simulink model "inverse_dynamic_with_pid"  (R2018a)
settings: Solver=ode45  StartTime=0.0  StopTime=3  RelTol=1e-3
libraries: simulink x6
settings Model: Creator=JORDAN  LastModifiedBy=JORDAN
settings DebuggingCC: LibraryContextMissingDiagnostic=warning
settings SFSimCC: SimUseLocalCustomCode=on
settings RTWCC: RTWUseLocalCustomCode=on

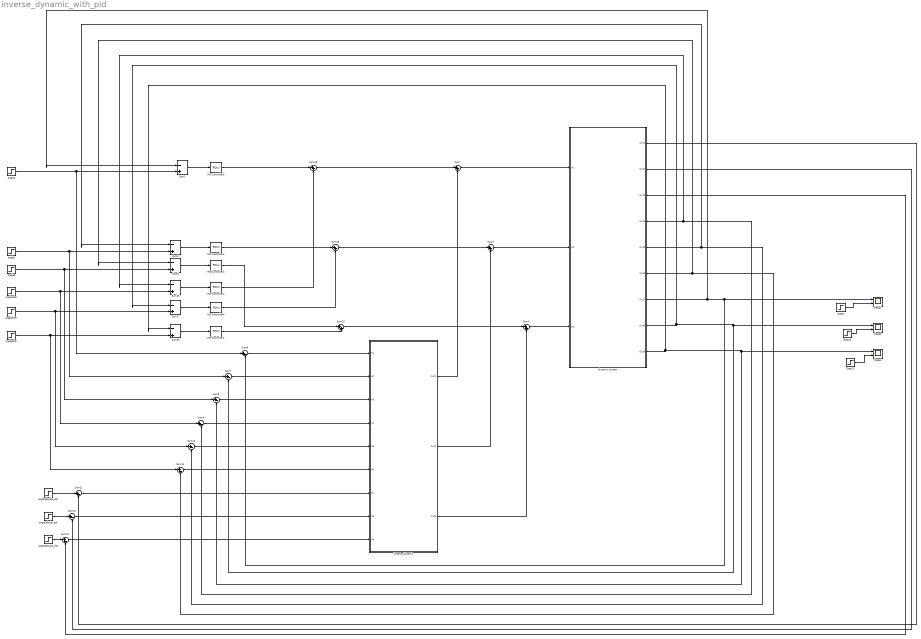
== system inverse_dynamic_with_pid ==
  PID Controller1 : simulink/Continuous/PID Controller  Controller=PD  Form=Parallel  TimeDomain=Continuous-time  SampleTime=-1  IntegratorMethod=Forward Euler  FilterMethod=Forward Euler  ControllerParametersSource=internal  P=75000  I=1  D=6000  UseFilter=on  N=7500  TunerSelectOption=Transfer Function Based (PID Tuner App)  InitialConditionSource=internal  InitialConditionForIntegrator=0  InitialConditionForFilter=0  DifferentiatorICPrevScaledInput=0  ExternalReset=none  TrackingMode=off  Kt=1  LimitOutput=off  UpperSaturationLimit=inf  LowerSaturationLimit=-inf  LinearizeAsGain=on  AntiWindupMode=none  Kb=1  POutMin=[]  POutMax=[]  IOutMin=[]  IOutMax=[]  DOutMin=[]  DOutMax=[]  NOutMin=[]  NOutMax=[]  SumOutMin=[]  SumOutMax=[]  SaturationOutMin=[]  SaturationOutMax=[]  PParamMin=[]  PParamMax=[]  IParamMin=[]  IParamMax=[]  DParamMin=[]  DParamMax=[]  NParamMin=[]  NParamMax=[]  KbParamMin=[]  KbParamMax=[]  KtParamMin=[]  KtParamMax=[]  KbOutMin=[]  KbOutMax=[]  KtOutMin=[]  KtOutMax=[]  IntegratorOutMin=[]  IntegratorOutMax=[]  FilterOutMin=[]  FilterOutMax=[]  SumI1OutMin=[]  SumI1OutMax=[]  SumI2OutMin=[]  SumI2OutMax=[]  SumI3OutMin=[]  SumI3OutMax=[]  SumDOutMin=[]  SumDOutMax=[]  DifferentiatorOutMin=[]  DifferentiatorOutMax=[]  FilterDiffOutCoefMin=[]  FilterDiffOutCoefMax=[]  ReciprocalOutMin=[]  ReciprocalOutMax=[]  SumDenOutMin=[]  SumDenOutMax=[]  SumNumOutMin=[]  SumNumOutMax=[]  DivideOutMin=[]  DivideOutMax=[]  IntegratorContinuousStateAttributes=''  IntegratorStateMustResolveToSignalObject=off  IntegratorRTWStateStorageClass=Auto  FilterContinuousStateAttributes=''  FilterStateMustResolveToSignalObject=off  FilterRTWStateStorageClass=Auto
  PID Controller2 : simulink/Continuous/PID Controller  Controller=PD  Form=Parallel  TimeDomain=Continuous-time  SampleTime=-1  IntegratorMethod=Forward Euler  FilterMethod=Forward Euler  ControllerParametersSource=internal  P=6000  I=1  D=0  UseFilter=on  N=100  TunerSelectOption=Transfer Function Based (PID Tuner App)  InitialConditionSource=internal  InitialConditionForIntegrator=0  InitialConditionForFilter=0  DifferentiatorICPrevScaledInput=0  ExternalReset=none  TrackingMode=off  Kt=1  LimitOutput=off  UpperSaturationLimit=inf  LowerSaturationLimit=-inf  LinearizeAsGain=on  AntiWindupMode=none  Kb=1  POutMin=[]  POutMax=[]  IOutMin=[]  IOutMax=[]  DOutMin=[]  DOutMax=[]  NOutMin=[]  NOutMax=[]  SumOutMin=[]  SumOutMax=[]  SaturationOutMin=[]  SaturationOutMax=[]  PParamMin=[]  PParamMax=[]  IParamMin=[]  IParamMax=[]  DParamMin=[]  DParamMax=[]  NParamMin=[]  NParamMax=[]  KbParamMin=[]  KbParamMax=[]  KtParamMin=[]  KtParamMax=[]  KbOutMin=[]  KbOutMax=[]  KtOutMin=[]  KtOutMax=[]  IntegratorOutMin=[]  IntegratorOutMax=[]  FilterOutMin=[]  FilterOutMax=[]  SumI1OutMin=[]  SumI1OutMax=[]  SumI2OutMin=[]  SumI2OutMax=[]  SumI3OutMin=[]  SumI3OutMax=[]  SumDOutMin=[]  SumDOutMax=[]  DifferentiatorOutMin=[]  DifferentiatorOutMax=[]  FilterDiffOutCoefMin=[]  FilterDiffOutCoefMax=[]  ReciprocalOutMin=[]  ReciprocalOutMax=[]  SumDenOutMin=[]  SumDenOutMax=[]  SumNumOutMin=[]  SumNumOutMax=[]  DivideOutMin=[]  DivideOutMax=[]  IntegratorContinuousStateAttributes=''  IntegratorStateMustResolveToSignalObject=off  IntegratorRTWStateStorageClass=Auto  FilterContinuousStateAttributes=''  FilterStateMustResolveToSignalObject=off  FilterRTWStateStorageClass=Auto
  PID Controller3 : simulink/Continuous/PID Controller  Controller=PD  Form=Parallel  TimeDomain=Continuous-time  SampleTime=-1  IntegratorMethod=Forward Euler  FilterMethod=Forward Euler  ControllerParametersSource=internal  P=150  I=1  D=0  UseFilter=on  N=100  TunerSelectOption=Transfer Function Based (PID Tuner App)  InitialConditionSource=internal  InitialConditionForIntegrator=0  InitialConditionForFilter=0  DifferentiatorICPrevScaledInput=0  ExternalReset=none  TrackingMode=off  Kt=1  LimitOutput=off  UpperSaturationLimit=inf  LowerSaturationLimit=-inf  LinearizeAsGain=on  AntiWindupMode=none  Kb=1  POutMin=[]  POutMax=[]  IOutMin=[]  IOutMax=[]  DOutMin=[]  DOutMax=[]  NOutMin=[]  NOutMax=[]  SumOutMin=[]  SumOutMax=[]  SaturationOutMin=[]  SaturationOutMax=[]  PParamMin=[]  PParamMax=[]  IParamMin=[]  IParamMax=[]  DParamMin=[]  DParamMax=[]  NParamMin=[]  NParamMax=[]  KbParamMin=[]  KbParamMax=[]  KtParamMin=[]  KtParamMax=[]  KbOutMin=[]  KbOutMax=[]  KtOutMin=[]  KtOutMax=[]  IntegratorOutMin=[]  IntegratorOutMax=[]  FilterOutMin=[]  FilterOutMax=[]  SumI1OutMin=[]  SumI1OutMax=[]  SumI2OutMin=[]  SumI2OutMax=[]  SumI3OutMin=[]  SumI3OutMax=[]  SumDOutMin=[]  SumDOutMax=[]  DifferentiatorOutMin=[]  DifferentiatorOutMax=[]  FilterDiffOutCoefMin=[]  FilterDiffOutCoefMax=[]  ReciprocalOutMin=[]  ReciprocalOutMax=[]  SumDenOutMin=[]  SumDenOutMax=[]  SumNumOutMin=[]  SumNumOutMax=[]  DivideOutMin=[]  DivideOutMax=[]  IntegratorContinuousStateAttributes=''  IntegratorStateMustResolveToSignalObject=off  IntegratorRTWStateStorageClass=Auto  FilterContinuousStateAttributes=''  FilterStateMustResolveToSignalObject=off  FilterRTWStateStorageClass=Auto
  PID Controller4 : simulink/Continuous/PID Controller  Controller=PD  Form=Parallel  TimeDomain=Continuous-time  SampleTime=-1  IntegratorMethod=Forward Euler  FilterMethod=Forward Euler  ControllerParametersSource=internal  P=1  I=1  D=0  UseFilter=on  N=100  TunerSelectOption=Transfer Function Based (PID Tuner App)  InitialConditionSource=internal  InitialConditionForIntegrator=0  InitialConditionForFilter=0  DifferentiatorICPrevScaledInput=0  ExternalReset=none  TrackingMode=off  Kt=1  LimitOutput=off  UpperSaturationLimit=inf  LowerSaturationLimit=-inf  LinearizeAsGain=on  AntiWindupMode=none  Kb=1  POutMin=[]  POutMax=[]  IOutMin=[]  IOutMax=[]  DOutMin=[]  DOutMax=[]  NOutMin=[]  NOutMax=[]  SumOutMin=[]  SumOutMax=[]  SaturationOutMin=[]  SaturationOutMax=[]  PParamMin=[]  PParamMax=[]  IParamMin=[]  IParamMax=[]  DParamMin=[]  DParamMax=[]  NParamMin=[]  NParamMax=[]  KbParamMin=[]  KbParamMax=[]  KtParamMin=[]  KtParamMax=[]  KbOutMin=[]  KbOutMax=[]  KtOutMin=[]  KtOutMax=[]  IntegratorOutMin=[]  IntegratorOutMax=[]  FilterOutMin=[]  FilterOutMax=[]  SumI1OutMin=[]  SumI1OutMax=[]  SumI2OutMin=[]  SumI2OutMax=[]  SumI3OutMin=[]  SumI3OutMax=[]  SumDOutMin=[]  SumDOutMax=[]  DifferentiatorOutMin=[]  DifferentiatorOutMax=[]  FilterDiffOutCoefMin=[]  FilterDiffOutCoefMax=[]  ReciprocalOutMin=[]  ReciprocalOutMax=[]  SumDenOutMin=[]  SumDenOutMax=[]  SumNumOutMin=[]  SumNumOutMax=[]  DivideOutMin=[]  DivideOutMax=[]  IntegratorContinuousStateAttributes=''  IntegratorStateMustResolveToSignalObject=off  IntegratorRTWStateStorageClass=Auto  FilterContinuousStateAttributes=''  FilterStateMustResolveToSignalObject=off  FilterRTWStateStorageClass=Auto
  PID Controller5 : simulink/Continuous/PID Controller  Controller=PD  Form=Parallel  TimeDomain=Continuous-time  SampleTime=-1  IntegratorMethod=Forward Euler  FilterMethod=Forward Euler  ControllerParametersSource=internal  P=1  I=1  D=0  UseFilter=on  N=100  TunerSelectOption=Transfer Function Based (PID Tuner App)  InitialConditionSource=internal  InitialConditionForIntegrator=0  InitialConditionForFilter=0  DifferentiatorICPrevScaledInput=0  ExternalReset=none  TrackingMode=off  Kt=1  LimitOutput=off  UpperSaturationLimit=inf  LowerSaturationLimit=-inf  LinearizeAsGain=on  AntiWindupMode=none  Kb=1  POutMin=[]  POutMax=[]  IOutMin=[]  IOutMax=[]  DOutMin=[]  DOutMax=[]  NOutMin=[]  NOutMax=[]  SumOutMin=[]  SumOutMax=[]  SaturationOutMin=[]  SaturationOutMax=[]  PParamMin=[]  PParamMax=[]  IParamMin=[]  IParamMax=[]  DParamMin=[]  DParamMax=[]  NParamMin=[]  NParamMax=[]  KbParamMin=[]  KbParamMax=[]  KtParamMin=[]  KtParamMax=[]  KbOutMin=[]  KbOutMax=[]  KtOutMin=[]  KtOutMax=[]  IntegratorOutMin=[]  IntegratorOutMax=[]  FilterOutMin=[]  FilterOutMax=[]  SumI1OutMin=[]  SumI1OutMax=[]  SumI2OutMin=[]  SumI2OutMax=[]  SumI3OutMin=[]  SumI3OutMax=[]  SumDOutMin=[]  SumDOutMax=[]  DifferentiatorOutMin=[]  DifferentiatorOutMax=[]  FilterDiffOutCoefMin=[]  FilterDiffOutCoefMax=[]  ReciprocalOutMin=[]  ReciprocalOutMax=[]  SumDenOutMin=[]  SumDenOutMax=[]  SumNumOutMin=[]  SumNumOutMax=[]  DivideOutMin=[]  DivideOutMax=[]  IntegratorContinuousStateAttributes=''  IntegratorStateMustResolveToSignalObject=off  IntegratorRTWStateStorageClass=Auto  FilterContinuousStateAttributes=''  FilterStateMustResolveToSignalObject=off  FilterRTWStateStorageClass=Auto
  PID Controller6 : simulink/Continuous/PID Controller  Controller=PD  Form=Parallel  TimeDomain=Continuous-time  SampleTime=-1  IntegratorMethod=Forward Euler  FilterMethod=Forward Euler  ControllerParametersSource=internal  P=337900  I=1  D=19000  UseFilter=on  N=6170  TunerSelectOption=Transfer Function Based (PID Tuner App)  InitialConditionSource=internal  InitialConditionForIntegrator=0  InitialConditionForFilter=0  DifferentiatorICPrevScaledInput=0  ExternalReset=none  TrackingMode=off  Kt=1  LimitOutput=off  UpperSaturationLimit=inf  LowerSaturationLimit=-inf  LinearizeAsGain=on  AntiWindupMode=none  Kb=1  POutMin=[]  POutMax=[]  IOutMin=[]  IOutMax=[]  DOutMin=[]  DOutMax=[]  NOutMin=[]  NOutMax=[]  SumOutMin=[]  SumOutMax=[]  SaturationOutMin=[]  SaturationOutMax=[]  PParamMin=[]  PParamMax=[]  IParamMin=[]  IParamMax=[]  DParamMin=[]  DParamMax=[]  NParamMin=[]  NParamMax=[]  KbParamMin=[]  KbParamMax=[]  KtParamMin=[]  KtParamMax=[]  KbOutMin=[]  KbOutMax=[]  KtOutMin=[]  KtOutMax=[]  IntegratorOutMin=[]  IntegratorOutMax=[]  FilterOutMin=[]  FilterOutMax=[]  SumI1OutMin=[]  SumI1OutMax=[]  SumI2OutMin=[]  SumI2OutMax=[]  SumI3OutMin=[]  SumI3OutMax=[]  SumDOutMin=[]  SumDOutMax=[]  DifferentiatorOutMin=[]  DifferentiatorOutMax=[]  FilterDiffOutCoefMin=[]  FilterDiffOutCoefMax=[]  ReciprocalOutMin=[]  ReciprocalOutMax=[]  SumDenOutMin=[]  SumDenOutMax=[]  SumNumOutMin=[]  SumNumOutMax=[]  DivideOutMin=[]  DivideOutMax=[]  IntegratorContinuousStateAttributes=''  IntegratorStateMustResolveToSignalObject=off  IntegratorRTWStateStorageClass=Auto  FilterContinuousStateAttributes=''  FilterStateMustResolveToSignalObject=off  FilterRTWStateStorageClass=Auto
  Step10 : Step  Time=0  SampleTime=0
  Step11 : Step  Time=0  SampleTime=0
  Step9 : Step  Time=0  SampleTime=0
  Sum{,3..4,18..20} (6 alike) : Sum  Inputs=|++
  Sum{1..2,5,15..17} (6 alike) : Sum  Inputs=|-+
  Sum{6..14} (9 alike) : Sum  Inputs=|+-
  angle1 : Step  SampleTime=0
  angle1dot : Step  Time=0  SampleTime=0
  angle1double_dot : Step  Time=0  SampleTime=0
  angle2 : Step  SampleTime=0
  angle2dot : Step  Time=0  SampleTime=0
  angle2doule_dot : Step  Time=0  SampleTime=0
  angle3 : Step  SampleTime=0
  angle3dot : Step  Time=0  SampleTime=0
  angle3double_dot : Step  Time=0  SampleTime=0
  dynamic system : Subsystem
  inverse_dynamic : Subsystem
  theta1 : Scope  NumInputPorts=2
  theta2 : Scope  NumInputPorts=2
  theta3 : Scope  NumInputPorts=2
  wires:
  inverse_dynamic/1(Out1) -> Sum/2
  inverse_dynamic/2(Out2) -> Sum3/2
  inverse_dynamic/3(Out3) -> Sum4/2
  angle1/1 -> Sum6/1, Sum1/2
  angle3/1 -> Sum5/2, Sum8/1
  angle2dot/1 -> Sum17/2, Sum14/1
  angle3dot/1 -> Sum12/1, Sum15/2
  angle1dot/1 -> Sum16/2, Sum9/1
  angle2/1 -> Sum2/2, Sum7/1
  angle1double_dot/1 -> Sum11/1
  angle2doule_dot/1 -> Sum10/1
  angle3double_dot/1 -> Sum13/1
  Sum6/1 -> inverse_dynamic/1(In1)
  Sum7/1 -> inverse_dynamic/2(In2)
  Sum8/1 -> inverse_dynamic/3(In3)
  Sum9/1 -> inverse_dynamic/4(In4)
  Sum14/1 -> inverse_dynamic/5(In5)
  Sum12/1 -> inverse_dynamic/6(In6)
  Sum11/1 -> inverse_dynamic/7(In7)
  Sum10/1 -> inverse_dynamic/8(In8)
  Sum13/1 -> inverse_dynamic/9(In9)
  Sum1/1 -> PID Controller5/1
  Sum2/1 -> PID Controller2/1
  Sum5/1 -> PID Controller3/1
  dynamic system/8(Out8) -> Sum17/1, theta2/1, Sum7/2
  dynamic system/9(Out9) -> theta3/1, Sum8/2, Sum15/1
  dynamic system/7(Out7) -> Sum1/1, theta1/1, Sum6/2
  dynamic system/5(Out5) -> Sum2/1, Sum14/2
  dynamic system/2(Out2) -> Sum10/2
  dynamic system/4(Out4) -> Sum16/1, Sum9/2
  Sum4/1 -> dynamic system/3(In3)
  dynamic system/3(Out3) -> Sum13/2
  dynamic system/6(Out6) -> Sum5/1, Sum12/2
  dynamic system/1(Out1) -> Sum11/2
  Sum3/1 -> dynamic system/2(In2)
  Sum/1 -> dynamic system/1(In1)
  Sum15/1 -> PID Controller1/1
  Sum17/1 -> PID Controller6/1
  Sum16/1 -> PID Controller4/1
  PID Controller5/1 -> Sum19/1
  PID Controller4/1 -> Sum19/2
  PID Controller2/1 -> Sum18/1
  PID Controller6/1 -> Sum18/2
  PID Controller3/1 -> Sum20/1
  PID Controller1/1 -> Sum20/2
  Sum19/1 -> Sum/1
  Sum18/1 -> Sum3/1
  Sum20/1 -> Sum4/1
  Step9/1 -> theta1/2
  Step10/1 -> theta2/2
  Step11/1 -> theta3/2

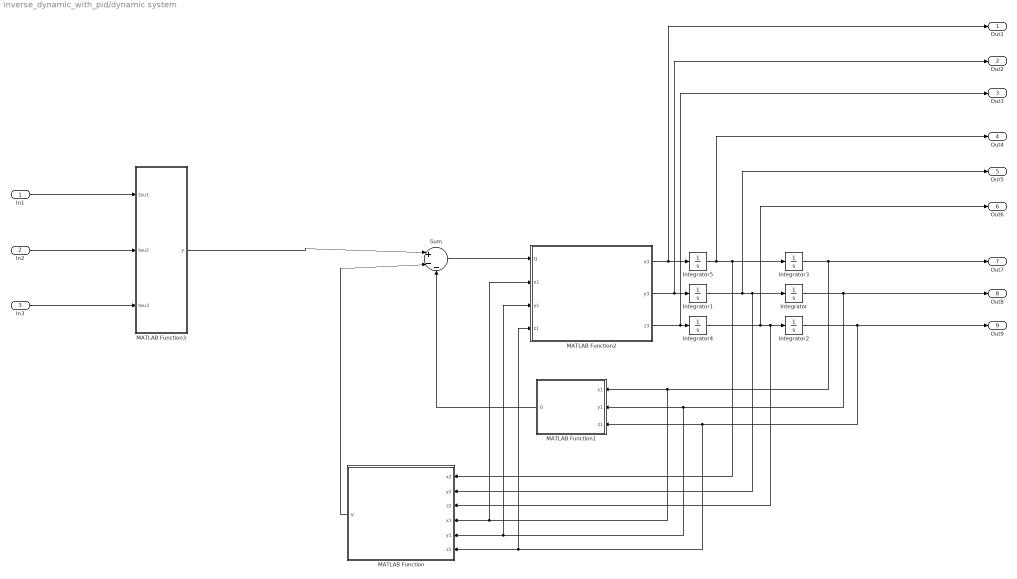
== system inverse_dynamic_with_pid/dynamic system ==
  In1 : Inport
  In2 : Inport  Port=2
  In3 : Inport  Port=3
  Integrator{,2..5} (5 alike) : Integrator
  Integrator1 : Integrator  InitialCondition=0.0000001
  MATLAB Function : MATLAB Function  TreatAsAtomicUnit=on
  MATLAB Function1 : MATLAB Function  TreatAsAtomicUnit=on
  MATLAB Function2 : MATLAB Function  TreatAsAtomicUnit=on
  MATLAB Function3 : MATLAB Function  TreatAsAtomicUnit=on
  Sum : Sum  Inputs=|+--
  Out1 : Outport
  Out2 : Outport  Port=2
  Out3 : Outport  Port=3
  Out4 : Outport  Port=4
  Out5 : Outport  Port=5
  Out6 : Outport  Port=6
  Out7 : Outport  Port=7
  Out8 : Outport  Port=8
  Out9 : Outport  Port=9
  wires:
  Integrator5/1 -> Out4/1, MATLAB Function/1(x2), Integrator3/1
  Integrator1/1 -> Out5/1, Integrator/1, MATLAB Function/2(y2)
  Integrator3/1 -> Out7/1, MATLAB Function2/2(x1), MATLAB Function/4(x1), MATLAB Function1/1(x1)
  MATLAB Function2/3(z3) -> Out3/1, Integrator4/1
  Integrator4/1 -> Out6/1, MATLAB Function/3(z2), Integrator2/1
  MATLAB Function2/2(y3) -> Out2/1, Integrator1/1
  Integrator/1 -> Out8/1, MATLAB Function2/3(y1), MATLAB Function/5(y1), MATLAB Function1/2(y1)
  MATLAB Function/1(V) -> Sum/2
  MATLAB Function2/1(x3) -> Out1/1, Integrator5/1
  MATLAB Function1/1(G) -> Sum/3
  In2/1 -> MATLAB Function3/2(tau2)
  In1/1 -> MATLAB Function3/1(tau1)
  Sum/1 -> MATLAB Function2/1(Q)
  Integrator2/1 -> Out9/1, MATLAB Function2/4(z1), MATLAB Function/6(z1), MATLAB Function1/3(z1)
  MATLAB Function3/1(y) -> Sum/1
  In3/1 -> MATLAB Function3/3(tau3)

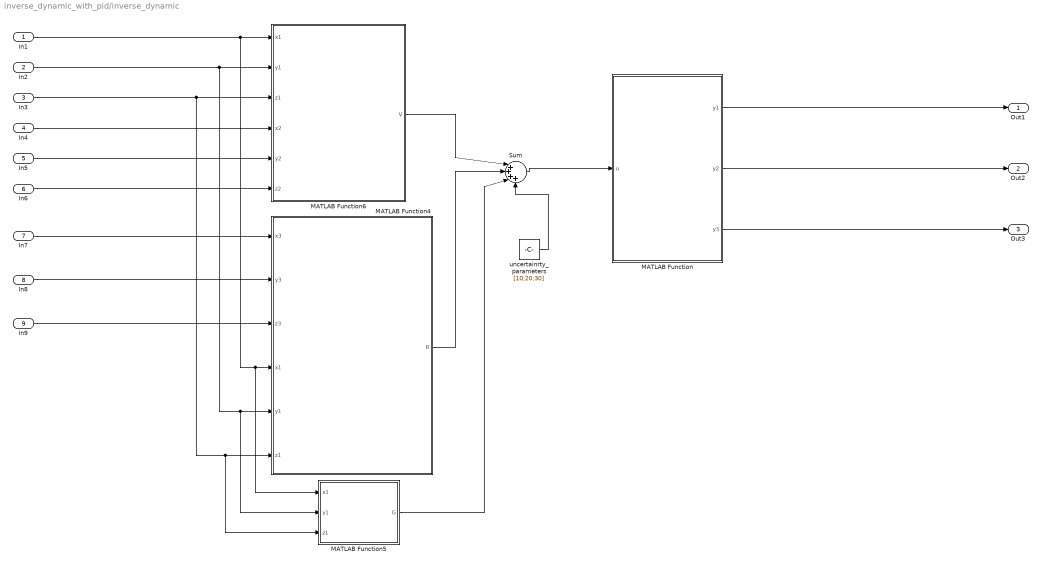
== system inverse_dynamic_with_pid/inverse_dynamic ==
  In1 : Inport
  In2 : Inport  Port=2
  In3 : Inport  Port=3
  In4 : Inport  Port=4
  In5 : Inport  Port=5
  In6 : Inport  Port=6
  In7 : Inport  Port=7
  In8 : Inport  Port=8
  In9 : Inport  Port=9
  MATLAB Function : MATLAB Function  TreatAsAtomicUnit=on
  MATLAB Function4 : MATLAB Function  TreatAsAtomicUnit=on
  MATLAB Function5 : MATLAB Function  TreatAsAtomicUnit=on
  MATLAB Function6 : MATLAB Function  TreatAsAtomicUnit=on
  Sum : Sum  Inputs=|++++
  uncertainrty_parameters : Constant  Value=[10;20;30]
  Out1 : Outport
  Out2 : Outport  Port=2
  Out3 : Outport  Port=3
  wires:
  MATLAB Function/1(y1) -> Out1/1
  MATLAB Function/2(y2) -> Out2/1
  In1/1 -> MATLAB Function5/1(x1), MATLAB Function4/4(x1), MATLAB Function6/1(x1)
  In2/1 -> MATLAB Function5/2(y1), MATLAB Function4/5(y1), MATLAB Function6/2(y1)
  In3/1 -> MATLAB Function5/3(z1), MATLAB Function4/6(z1), MATLAB Function6/3(z1)
  MATLAB Function4/1(R) -> Sum/2
  MATLAB Function6/1(V) -> Sum/1
  MATLAB Function5/1(G) -> Sum/3
  Sum/1 -> MATLAB Function/1(u)
  In5/1 -> MATLAB Function6/5(y2)
  In6/1 -> MATLAB Function6/6(z2)
  MATLAB Function/3(y3) -> Out3/1
  In4/1 -> MATLAB Function6/4(x2)
  In7/1 -> MATLAB Function4/1(x3)
  In9/1 -> MATLAB Function4/3(z3)
  In8/1 -> MATLAB Function4/2(y3)
  uncertainrty_parameters/1 -> Sum/4

== matlab function inverse_dynamic_with_pid/dynamic system/MATLAB Function ==
  data: x2 input; V output size=3*1; y2 input; z2 input; x1 input; y1 input; z1 input
function V = vmatrix(x2,y2,z2,x1,y1,z1)
m2=3; 
m3=2;
l2=5; 
l3=3;
r=10;
V=[(-0.25*m3*(r^2)*sin(y1)*cos(y1)*x2*z2)-((1/6)*m2*l2^2*cos(y1)*sin(y1)*x2*y2)+((2/3)*m3*l3^2*cos(y1)*cos(z1)*sin(z1-y1)*x2*y2)+(0.5*m3*(r^2)*sin(y1-z1)*cos(y1-z1)*x2*y2)+((3/4)*m2*(r^2)*sin(y1)*cos(y1)*x2*y2)+((1/6)*m3*l3^2*sin(y1)*sin(z1-x1)*x2*y2)+(0.5*m3*l3^2*sin(y1)*sin(z1)*sin(z1-y1)*x2*y2)+(0.5*m3*l2*l3*cos(y1)*cos(y1-z1)*x2)+(m3*l2*l3*sin(y1)*sin(y1)*sin(z1)*x2*y2)-(0.25*m2*(r^2)*cos(y1)*sin(y1)*x2*y2)-(m3*l2*l3*cos(y1)*sin(y1)*cos(z1)*x2*y2)-(0.5*m2*l2^2*cos(y1)*sin(y1)*x2*y2)+(m3*l2*l3*cos(y1)*sin(z1-y1)*x2*y2)+(m3*l2^2*cos(y1)*cos(y1)*x2)+(2*m3*l2^2*cos(y1)*sin(y1)*x2*y2) ; 
    (-0.25*m2*(r^2)*cos(y1)*sin(y1)*(x2^2))+((1/12)*m2*l2^2*sin(y1)*cos(y1)*(x2^2))+(0.25*m3*(r^2)*cos(y1-z1)*sin(z1-y1)*(x2^2))-((1/3)*m3*l3^2*cos(y1-z1)*sin(z1-y1)*(x2^2))-(0.25*m3*l3^2*z2)+(0.5*m3*l3*l2*cos(y1)*cos(z1-y1)*(x2^2))-(0.5*m3*l3*l2*sin(z1)*(y2^2))+(0.25*m2*l2^2*sin(y1)*cos(y1)*(x2^2))+(0.5*m3*l3*l2*sin(z1)*cos(y1-z1)*(x2^2))+(0.5*m3*l3*l2*sin(z1)*(z2^2))+(0.5*m3*l3*l2*sin(z1)*(y2^2))-(m3*l3*l2*sin(z1)*y2*z2)+(m3*l2^2*cos(y1)*sin(y1)*cos(z1-y1)*(x2^2))-(0.5*m3*l3*l2*cos(z1)*cos(y1-z1)*sin(z1-y1)*(x2^2))+(m3*l2^2*cos(y1)*cos(z1)*cos(z1-y1)*(x2^2)) ; 
    (-0.25*m3*(r^2)*cos(y1-z1)*sin(z1-y1)*(x2^2))+((1/3)*m3*l3^2*cos(y1-z1)*sin(z1-y1)*(x2^2))+(0.25*m3*l3^2*z2)-(0.5*m3*l3*l2*cos(y1)*cos(z1-y1)*(x2^2))+(0.5*m3*l3*l2*sin(z1)*(y2^2))];

== matlab function inverse_dynamic_with_pid/inverse_dynamic/MATLAB Function ==
  data: u input; y1 output; y2 output; y3 output
function [y1,y2,y3] = tau_matrix(u)

y1=u(1,1);
y2=u(2,1);
y3=u(3,1);

== matlab function inverse_dynamic_with_pid/dynamic system/MATLAB Function1 ==
  data: x1 input; G output; y1 input; z1 input
function G = gravity(x1,y1,z1)
g=10;
m2=3;
m3=2;
l2=5;
l3=3;
r=10;
G=[0 ; (-0.5*m3*l2*cos(y1-z1)*g)-(0.5*m2*l2*cos(y1)*g)+(m3*l2*sin(z1)*sin(y1-z1)*g) ; (0.5*m3*l3*cos(y1-z1)*g)]

== matlab function inverse_dynamic_with_pid/dynamic system/MATLAB Function2 ==
  data: Q input; x3 output; y3 output; z3 output; x1 input; y1 input; z1 input
function  [x3,y3,z3]= mass_matrix(Q,x1,y1,z1)
m1=5;
m2=3;
m3=2;
l2=5;
l3=3;
r=10;
p=[(0.25*m2*(r^2)*((2*sin(y1)*sin(y1))+(cos(y1)*cos(y1))))+(0.25*m3*(r^2)*((2*sin(z1-y1)*sin(z1-y1))+(cos(z1-y1)*cos(z1-y1))))+((1/12)*m3*sin(y1)*sin(z1)*cos(y1-z1)*(l2^2+3*l3^2))+((1/6)*m3*l3*cos(y1)*cos(y1-z1)*(2*l3*cos(z1)+3*l2))+(0.5*m1*r)+((1/3)*m2*l2^2*cos(y1)*cos(y1)) 0 0 ; 
0 ((1/12)*m2*((3*r^2)+l2^2))+(0.25*m3*(r^2+l3^2))+(m3*l3*l2*cos(z1)+(l2^2*(0.25*m2+m3))) (-(1/12)*m3*((3*r^2)+4*l3^2))-(0.5*m3*l3*l2*cos(z1)) ; 
0 (-(1/12)*m3*(3*r^2+4*l3^2))-(0.5*m3*l3*l2*cos(z1)) ((1/12)*m3*(3*r^2+l3^2))]
R=inv(p)*Q
x3=R(1,1);
y3=R(2,1);
z3=R(3,1);

== matlab function inverse_dynamic_with_pid/inverse_dynamic/MATLAB Function4 ==
  data: x3 input; y3 input; z3 input; R output; x1 input; y1 input; z1 input
function R = mass_matrix(x3,y3,z3,x1,y1,z1)
m1=5;
m2=3;
m3=2;
l2=5;
l3=3;
r=10;
p=[(0.25*m2*(r^2)*((2*sin(y1)*sin(y1))+(cos(y1)*cos(y1))))+(0.25*m3*(r^2)*((2*sin(z1-y1)*sin(z1-y1))+(cos(z1-y1)*cos(z1-y1))))+((1/12)*m3*sin(y1)*sin(z1)*cos(y1-z1)*(l2^2+3*l3^2))+((1/6)*m3*l3*cos(y1)*cos(y1-z1)*(2*l3*cos(z1)+3*l2))+(0.5*m1*r)+((1/3)*m2*l2^2*cos(y1)*cos(y1)) 0 0 ; 
0 ((1/12)*m2*((3*r^2)+l2^2))+(0.25*m3*(r^2+l3^2))+(m3*l3*l2*cos(z1)+(l2^2*(0.25*m2+m3))) (-(1/12)*m3*((3*r^2)+4*l3^2))-(0.5*m3*l3*l2*cos(z1)) ; 
0 (-(1/12)*m3*(3*r^2+4*l3^2))-(0.5*m3*l3*l2*cos(z1)) ((1/12)*m3*(3*r^2+l3^2))]
n=[x3;y3;z3];
R=p*n

== matlab function inverse_dynamic_with_pid/inverse_dynamic/MATLAB Function5 ==
  data: x1 input; G output; y1 input; z1 input
function G = gravity(x1,y1,z1)
g=10;
m2=3;
m3=2;
l2=5;
l3=3;
r=10;
G=[0 ; (-0.5*m3*l2*cos(y1-z1)*g)-(0.5*m2*l2*cos(y1)*g)+(m3*l2*sin(z1)*sin(y1-z1)*g) ; (0.5*m3*l3*cos(y1-z1)*g)]

== matlab function inverse_dynamic_with_pid/dynamic system/MATLAB Function3 ==
  data: tau1 input; y output; tau2 input; tau3 input
function y = tau_matix(tau1,tau2,tau3)
y=[tau1;tau2;tau3];

== matlab function inverse_dynamic_with_pid/inverse_dynamic/MATLAB Function6 ==
  data: x1 input; y1 input; z1 input; x2 input; V output size=3*1; y2 input; z2 input
function V = vmatrix(x1,y1,z1,x2,y2,z2)
m2=3; 
m3=2;
l2=5; 
l3=3;
r=10;
V=[(-0.25*m3*(r^2)*sin(y1)*cos(y1)*x2*z2)-((1/6)*m2*l2^2*cos(y1)*sin(y1)*x2*y2)+((2/3)*m3*l3^2*cos(y1)*cos(z1)*sin(z1-y1)*x2*y2)+(0.5*m3*(r^2)*sin(y1-z1)*cos(y1-z1)*x2*y2)+((3/4)*m2*(r^2)*sin(y1)*cos(y1)*x2*y2)+((1/6)*m3*l3^2*sin(y1)*sin(z1-x1)*x2*y2)+(0.5*m3*l3^2*sin(y1)*sin(z1)*sin(z1-y1)*x2*y2)+(0.5*m3*l2*l3*cos(y1)*cos(y1-z1)*x2)+(m3*l2*l3*sin(y1)*sin(y1)*sin(z1)*x2*y2)-(0.25*m2*(r^2)*cos(y1)*sin(y1)*x2*y2)-(m3*l2*l3*cos(y1)*sin(y1)*cos(z1)*x2*y2)-(0.5*m2*l2^2*cos(y1)*sin(y1)*x2*y2)+(m3*l2*l3*cos(y1)*sin(z1-y1)*x2*y2)+(m3*l2^2*cos(y1)*cos(y1)*x2)+(2*m3*l2^2*cos(y1)*sin(y1)*x2*y2) ; 
    (-0.25*m2*(r^2)*cos(y1)*sin(y1)*(x2^2))+((1/12)*m2*l2^2*sin(y1)*cos(y1)*(x2^2))+(0.25*m3*(r^2)*cos(y1-z1)*sin(z1-y1)*(x2^2))-((1/3)*m3*l3^2*cos(y1-z1)*sin(z1-y1)*(x2^2))-(0.25*m3*l3^2*z2)+(0.5*m3*l3*l2*cos(y1)*cos(z1-y1)*(x2^2))-(0.5*m3*l3*l2*sin(z1)*(y2^2))+(0.25*m2*l2^2*sin(y1)*cos(y1)*(x2^2))+(0.5*m3*l3*l2*sin(z1)*cos(y1-z1)*(x2^2))+(0.5*m3*l3*l2*sin(z1)*(z2^2))+(0.5*m3*l3*l2*sin(z1)*(y2^2))-(m3*l3*l2*sin(z1)*y2*z2)+(m3*l2^2*cos(y1)*sin(y1)*cos(z1-y1)*(x2^2))-(0.5*m3*l3*l2*cos(z1)*cos(y1-z1)*sin(z1-y1)*(x2^2))+(m3*l2^2*cos(y1)*cos(z1)*cos(z1-y1)*(x2^2)) ; 
    (-0.25*m3*(r^2)*cos(y1-z1)*sin(z1-y1)*(x2^2))+((1/3)*m3*l3^2*cos(y1-z1)*sin(z1-y1)*(x2^2))+(0.25*m3*l3^2*z2)-(0.5*m3*l3*l2*cos(y1)*cos(z1-y1)*(x2^2))+(0.5*m3*l3*l2*sin(z1)*(y2^2))];
